simulink model "simulated_physical_reactor_v4_isolated"  (R2023a)
settings: Solver=FixedStepAuto  StartTime=0.0  StopTime=500  FixedStep=ts  RelTol=1e-3
values from neighbouring files (symbols this model uses):
  actionDelay = 10    [MainCode.m]
  buffer = 10    [MainCode.m]
  C0_attack_c = 0    [MainCode.m]
  C0_noise = 1    [MainCode.m]
  C0_post_attack = 0    [MainCode.m]
  C0_post_attack_val = -.25    (= -0.25)    [MainCode.m]
  Ccell0 = cell0 / v_cell    (= 15384.6153846)    [MainCode.m]
  CG0 = 185    [MainCode.m]
  CG_attack_c = 55    [MainCode.m]
  CG_attack_time = 175    [MainCode.m]
  CG_fake_failure = 0    [MainCode.m]
  CG_fake_failure_noise = 8    [MainCode.m]
  CG_increase_b = 0    [MainCode.m]
  CG_increase_rate = 2    [MainCode.m]
  cg_noGrowth = 10    [MainCode.m]
  CG_noise = 1    [MainCode.m]
  CG_post_attack = 1    [MainCode.m]
  CG_post_attack_val = .25    (= 0.25)    [MainCode.m]
  CG_ramp_attack = 1    [MainCode.m]
  CG_ramp_time = 125    [MainCode.m]
  CG_target = 50    [MainCode.m]
  CM = 4    [MainCode.m]
  CO0 = .245    (= 0.245)    [MainCode.m]
  CO_attack_time = 80    [MainCode.m]
  CO_fake_failure = 0    [MainCode.m]
  CO_fake_failure_mean = .08    (= 0.08)    [MainCode.m]
  CO_fake_failure_noise = .005    (= 0.005)    [MainCode.m]
  CO_ramp_attack = 0    [MainCode.m]
  CO_ramp_time = 100    [MainCode.m]
  count_thresh = 3    [MainCode.m]
  F_fresh_max = 25    [MainCode.m]
  F_net = F_fresh_start + F_recycle_start    (= 334.8)    [MainCode.m]
  flowrateNoiseActive = 0    [MainCode.m]
  flowrateNoiseVal = 0.5 / 100    (= 0.005)    [MainCode.m]
  fresh_attack = 0    [MainCode.m]
  fresh_attack_time = 70    [MainCode.m]
  fresh_attack_val = .1    (= 0.1)    [MainCode.m]
  freshPump_fail_time = 30    [MainCode.m]
  freshPump_failure = 0    [MainCode.m]
  freshPump_response_increases = 2    [MainCode.m]
  freshPump_response_window = 10    [MainCode.m]
  g_failure_start_t = 80    [MainCode.m]
  g_fault_wait_time = 10    [MainCode.m]
  g_flowrate_control_windowsize = 10    [MainCode.m]
  g_lownoise_val = 1.25    [MainCode.m]
  g_numpoints_fail = g_standdev_window_size+1    (= 16)    [MainCode.m]
  g_numpoints_low = 4    [MainCode.m]
  g_prob_arraylen = 15    [MainCode.m]
  g_prob_count = 6    [MainCode.m]
  g_prob_thresh = .45    (= 0.45)    [MainCode.m]
  g_standdev_window_size = 15    [MainCode.m]
  g_standev_tol = 7    [MainCode.m]
  glucose_fail_noise = 10    [MainCode.m]
  glucosesensor_failure = 0    [MainCode.m]
  lowConc_controller_onState = 1    [MainCode.m]
  mean_noise_C0 = 0    [MainCode.m]
  mean_noise_CG = 0    [MainCode.m]
  mu_max = 0.0251    [MainCode.m]
  n_size = t_window/ts    (= 2.5)    [MainCode.m]
  n_size_CG = n_size    (= 2.5)    [MainCode.m]
  o2_alpha = .20    (= 0.2)    [MainCode.m]
  o2_fail_mean = .008    (= 0.008)    [MainCode.m]
  o2_fail_noise = .005    (= 0.005)    [MainCode.m]
  o2_fail_time = 50    [MainCode.m]
  o2_fault_halfrange = .01    (= 0.01)    [MainCode.m]
  o2_fault_numpoints = 5    [MainCode.m]
  o2_lownoise_val = .0008    (= 0.0008)    [MainCode.m]
  o2_movingaverage_window = 10    [MainCode.m]
  o2_numpoints_low = 6    [MainCode.m]
  o2_prob_arraylen = 10    [MainCode.m]
  o2_prob_count = 6    [MainCode.m]
  o2_prob_thresh = .45    (= 0.45)    [MainCode.m]
  o2sensor_failure = 0    [MainCode.m]
  OCR = 2.8e-11    [MainCode.m]
  p_thresh = .4    (= 0.4)    [MainCode.m]
  rec_attack = 0    [MainCode.m]
  rec_attack_time = 50    [MainCode.m]
  rec_attack_val = 120    [MainCode.m]
  recPump_drop_val = .02    (= 0.02)    [MainCode.m]
  recPump_fail_time = 30    [MainCode.m]
  recPump_failure = 0    [MainCode.m]
  recPump_rollingavg_samples_buildup = 10    [MainCode.m]
  recPump_smallDrop_size = 0.006    [MainCode.m]
  stdev_noise_C0 = .002    (= 0.002)    [MainCode.m]
  stdev_noise_CG = 3.5    [MainCode.m]
  t_crit_CG = .7    (= 0.7)    [MainCode.m]
  ts = 1    [MainCode.m]
  V = 65.0    (= 65)    [MainCode.m]
  v_cell = 65    [MainCode.m]
  YGC = 155 * 10^-6    (= 0.000155)    [MainCode.m]
undefined symbols (not defined in the file or in its folder): DiscIntNeverNeededParam, recPump_numDrops_waitTime, recPump_rollingavg_numDrops
libraries: simulink x16, sldrtlib x11, dspstat3 x8, aerolibanimutils x1
(part 3 of 3)

== matlab function simulated_physical_reactor_v4_isolated/Attack and Fault Detection System1/Recycle Pump Fault Detection/MATLAB Function ==
  data: dnr input; new_flowrate_commanded input; RecyclePumpFail output; oxygen_sensor input; samples_to_wait input; numDrops input; rolling_avg_samples_wait input; o2_rollavg_drop_spec input; large_drop_val input; delta_o2_out output; rolling_avg_out output
function [RecyclePumpFail,delta_o2_out, rolling_avg_out] = noRecycleResponse(dnr, new_flowrate_commanded, oxygen_sensor, samples_to_wait,numDrops, rolling_avg_samples_wait, o2_rollavg_drop_spec, large_drop_val)

%%%%%%% initilizing memory variables
persistent prevFlowrate;
persistent wait_count2;
persistent oxygenDecreasesCount;
persistent prevOxygen;
persistent large_drop_occurred;
persistent o2_rolling_average;
persistent prev_o2_rolling_average;
persistent after_waited_samples_wait;
persistent recyclePumpFailure;

if isempty(prevFlowrate)
    prevFlowrate = new_flowrate_commanded;
end

if isempty(oxygenDecreasesCount)
    oxygenDecreasesCount = 0;
end

if isempty(recyclePumpFailure)
    recyclePumpFailure = 0;
end

if isempty(after_waited_samples_wait)
    after_waited_samples_wait = 0;
end

if isempty(o2_rolling_average)
    o2_rolling_average = 0;
end

if isempty(prev_o2_rolling_average)
    prev_o2_rolling_average = 0;
end

if isempty(large_drop_occurred)
    large_drop_occurred = 0;
end

if isempty(prevOxygen)
    prevOxygen = oxygen_sensor;
end

if isempty(wait_count2)
    wait_count2 = 0;
end

if(dnr==0)

    %if the drop is large enough, triggered the large_drop condition
    %keep large drop toggled if previously toggled
    %if the net flowrate has dropped, it may be attributed to that
    if ((abs(oxygen_sensor - prevOxygen)>large_drop_val || large_drop_occurred==1) && new_flowrate_commanded==prevFlowrate)
        large_drop_occurred = 1;
        %initialize the rolling average
        o2_rolling_average = oxygen_sensor;
    else
        large_drop_occurred = 0;
    end

    if (large_drop_occurred==1)
        %update rolling average
        o2_rolling_average = (o2_rolling_average + oxygen_sensor) / 2;
        wait_count2 = wait_count2+1;
        if (wait_count2>=samples_to_wait && rolling_avg_samples_wait>=after_waited_samples_wait)
            if (prev_o2_rolling_average > (o2_rolling_average+o2_rollavg_drop_spec))
                oxygenDecreasesCount = oxygenDecreasesCount + 1;
                %if the number of decreases enough, triggered the fault
                if (oxygenDecreasesCount>=numDrops)
                    recyclePumpFailure=1;
                end
            end
            %if its waiting long enough and the drops havent happened,
            %false alarm, reset everything
            if (after_waited_samples_wait >= rolling_avg_samples_wait)
                large_drop_occurred = 0;
                wait_count2 = 0;
                after_waited_samples_wait = 0;
                oxygenDecreasesCount = 0;
                o2_rolling_average = 0;
                prev_o2_rolling_average = 0; %#ok<NASGU>
            end
            after_waited_samples_wait = after_waited_samples_wait + 1;
        end
        prev_o2_rolling_average = o2_rolling_average;
    end

    %%temp debug
    delta_o2_out = abs(oxygen_sensor - prevOxygen);
    rolling_avg_out = o2_rolling_average;
    %%

    prevOxygen = oxygen_sensor;

    RecyclePumpFail = recyclePumpFailure;
else
    RecyclePumpFail = 0;
    delta_o2_out=0;
    rolling_avg_out=0;
end

== matlab function simulated_physical_reactor_v4_isolated/Attack and Fault Detection System1/Steady State Detection System1/MATLAB Function2 ==
  data: P_loop_in input; P_loop_out output; ABG input; P output; x input; n input; t_crit input; run_ss_func output
% R. R. Rhinehart, Automated steady and transient state identification in
% noisy processes, in Proceedings of the American Control Conference, 2013,
% no. June 2013, pp. 4477–4493.
%
% Section V

function [P_loop_out, P, run_ss_func]= ssd(P_loop_in, ABG, x, n, t_crit)

if x==0
    P = 0;
    P_loop_out = 0;
    run_ss_func = false;

elseif ABG == 1
    P_loop_out = P_loop_in;
    P = P_loop_in;

    run_ss_func = false;

else
    run_ss_func = true;

    P_array = zeros(length(x),1);

    if n > length(x)
        n = length(x);
    end

    k = 1;
    should_break = 0;
    while 1
        from = k;
        to = from + n - 1;

        if to > length(x)
            to = length(x);
            n = to -from  + 1;
            should_break = 1;
        end

        x_active = x(from:to);

        % By first differencing xt it is possible to unbiasedly1 estimate the slope
        % m of the drift component mt as the arithmetic average of xt − xt−1 with
        % n sampled values of xt in the window which areequally spaced in time
        % i.e., given a uniform sampling period or cycle.
        m = 0;
        for t = 2 : n
            m = m + (x_active(t)-x_active(t-1));
        end
        m = m/n;

        % eq. 3
        mu = (sum(x_active) - sum(1:n)*m)/n;

        % eq. 4
        sd = 0;
        for t = 1 : n
            sd = sd + (x_active(t) - m*t-mu)^2;
        end
        sd = sqrt(sd/(n-2));

        % eq. 5
        y = 0;
        for t = 1 : n
            if abs(x_active(t)-mu) <= t_crit * sd
                y = y + 1;
            end
        end
        y = y/n;

        P_array(from:to,1) = y;

        if should_break == 1
            break;
        end

        k = k + n;
    end
    P = mean(P_array);
    P_loop_out = P;

end

== matlab function simulated_physical_reactor_v4_isolated/CO Attack System/MATLAB Function2 ==
  data: o2_in input; o2_out output; o2_noise input; o2_const input; isFailed input
function o2_out = o2_failure(o2_in, o2_noise, o2_const, isFailed)

if isFailed == 0
    o2_out = o2_in;
else
    o2_out = normrnd(o2_const,o2_noise);
end

== matlab function simulated_physical_reactor_v4_isolated/Attack and Fault Detection System1/Steady State Detection System1/MATLAB Function3 ==
  data: new_count output; SS_prev input; count input; count_thresh input; run_func input; p input; isSteadyState output; p_thresh input
function [new_count, isSteadyState]= fcn(SS_prev,count, count_thresh, run_func, p, p_thresh)



if run_func == true
    if SS_prev == 1 %last state WAS steady
        if p>p_thresh %still SS
            new_count = 0;
        else %changed to notSS
            new_count = count + 1;
        end
    else %last state was notSS
        if p<p_thresh %still notSS
            new_count = 0;
        else %changed to SS
            new_count = count + 1;
        end
    end
    if new_count >= count_thresh
        if SS_prev == 1
            isSteadyState = 0;
        else
            isSteadyState = 1;
        end
    else
        isSteadyState = SS_prev;
    end
else
    new_count = count;
    isSteadyState = SS_prev;
end





















%     if SS_temp_in==0
%         if p<p_thresh
%             isSteadyState = 0;
%             SS_temp_out = 0;
%         else %p > p_thresh
%             isSteadyState = 0;
%             SS_temp_out = 2;
%         end
% 
%     elseif SS_temp_in == 2
%         if p>p_thresh
%             isSteadyState = 1;
%             SS_temp_out = 1;
%         else %p < p_thresh
%             isSteadyState = 0;
%             SS_temp_out = 0;
%         end
%     else %SS_temp_in == 1
%         if p>p_thresh
%             isSteadyState = 1;
%             SS_temp_out = 1;
%         else %p < p_thresh
%             isSteadyState = 1;
%             SS_temp_out = 2;
%         end
%         
%     end
%     
% 
% else
%     isSteadyState = isSteadyState_loop_in;
%     SS_temp_out = SS_temp_in;
% end
% 
% isSteadyState_loop_out = isSteadyState;
% 
% whatLoop_in_was = isSteadyState_loop_in;
% whattempinwas = SS_temp_in;

== matlab function simulated_physical_reactor_v4_isolated/Attack and Fault Detection System1/Steady State Detection System1/MATLAB Function4 ==
  data: input input; ABG output; n_size input
function ABG = fcn(input, n_size)

if mod(input,n_size)==0
    ABG = -1;
else
    ABG = 1;
end

== matlab function simulated_physical_reactor_v4_isolated/Fresh Flowrate Fault System/MATLAB Function ==
  data: in_flow input; out_flow output; fault_on input; time input; fault_time input
function out_flow = fcn(in_flow, fault_on, time, fault_time)

if (fault_on==1 && time>fault_time)
    out_flow = 0;
else
    out_flow = in_flow;
end

== matlab function simulated_physical_reactor_v4_isolated/Recycle Flowrate Fault System/MATLAB Function ==
  data: in_flow input; out_flow output; fault_on input; time input; fault_time input
function out_flow = fcn(in_flow, fault_on, time, fault_time)

if (fault_on==1 && time>fault_time)
    out_flow = 0;
else
    out_flow = in_flow;
end

== matlab function simulated_physical_reactor_v4_isolated/Glucose sensor failure/MATLAB Function ==
  data: glucose_in input; glucoseOut output; glucose_noise input; isFailed input
function glucoseOut = glucose_failure(glucose_in, glucose_noise, isFailed)

if isFailed == 0
    glucoseOut = glucose_in;
else
    r = normrnd(0,glucose_noise);
    glucoseOut = glucose_in + r;
end

== matlab function simulated_physical_reactor_v4_isolated/recycle or fresh medium1 ==
  data: fresh_flowrate input; recycled_flowrate input; CG0 input; CG_recycled input; CG_inlet output; total_flowrate output
function [CG_inlet, total_flowrate]  = isNewFluid(fresh_flowrate, recycled_flowrate, CG0, CG_recycled)

%net flowrate into reactor is fresh+recycle rates
total_flowrate = fresh_flowrate + recycled_flowrate;

%glucose concentration is sum of each fluid stream's concentrations
CG_inlet = ((fresh_flowrate*CG0) + (recycled_flowrate*CG_recycled)) / total_flowrate;
